simulink model "lab6sim"  (R2020a)
settings: Solver=VariableStepAuto  StartTime=0.0  StopTime=30  RelTol=1e-3
undefined symbols (not defined in the file or in its folder): den1, den2, den3, num1, num2, num3
settings Model: Creator=ariana  LastModifiedBy=ariana

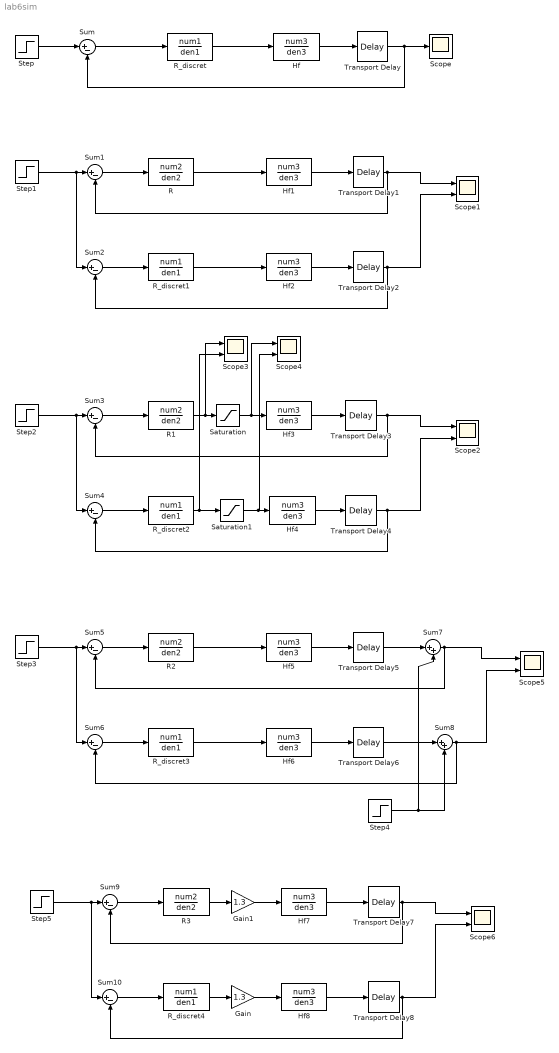
== system lab6sim ==
  Gain : Gain  Gain=1.3
  Gain1 : Gain  Gain=1.3
  Hf{,1..8} (9 alike) : TransferFcn  Numerator=num3  Denominator=den3
  R{,1..3} (4 alike) : TransferFcn  Numerator=num2  Denominator=den2
  R_discret{,1..4} (5 alike) : DiscreteTransferFcn  Numerator=num1  Denominator=den1  SampleTime=0.005
  Saturation : Saturate  UpperLimit=10  LowerLimit=0
  Saturation1 : Saturate  UpperLimit=10  LowerLimit=0
  Scope : Scope
  Scope{1..6} (6 alike) : Scope  NumInputPorts=2
  Step{,1..3,5} (5 alike) : Step  Time=0  After=20  SampleTime=0
  Step4 : Step  Time=10  After=5  SampleTime=0
  Sum{,1..6,9..10} (9 alike) : Sum  Inputs=|+-
  Sum7 : Sum  Inputs=|++
  Sum8 : Sum  Inputs=|++
  Transport Delay{,1..8} (9 alike) : TransportDelay  DelayTime=0.8
  wires:
  Step/1 -> Sum/1
  Sum/1 -> R_discret/1
  R_discret/1 -> Hf/1
  Hf/1 -> Transport Delay/1
  Transport Delay/1 -> Sum/2, Scope/1
  Step1/1 -> Sum2/1, Sum1/1
  Sum1/1 -> R/1
  Sum2/1 -> R_discret1/1
  R/1 -> Hf1/1
  R_discret1/1 -> Hf2/1
  Hf1/1 -> Transport Delay1/1
  Hf2/1 -> Transport Delay2/1
  Transport Delay1/1 -> Sum1/2, Scope1/1
  Transport Delay2/1 -> Sum2/2, Scope1/2
  Hf4/1 -> Transport Delay4/1
  Transport Delay3/1 -> Sum3/2, Scope2/1
  Transport Delay4/1 -> Sum4/2, Scope2/2
  Step2/1 -> Sum4/1, Sum3/1
  Hf3/1 -> Transport Delay3/1
  Sum3/1 -> R1/1
  R_discret2/1 -> Scope3/2, Saturation1/1
  Sum4/1 -> R_discret2/1
  R1/1 -> Scope3/1, Saturation/1
  Saturation1/1 -> Scope4/2, Hf4/1
  Saturation/1 -> Scope4/1, Hf3/1
  Sum5/1 -> R2/1
  Hf5/1 -> Transport Delay5/1
  Sum6/1 -> R_discret3/1
  Step3/1 -> Sum6/1, Sum5/1
  R2/1 -> Hf5/1
  R_discret3/1 -> Hf6/1
  Transport Delay5/1 -> Sum7/1
  Hf6/1 -> Transport Delay6/1
  Sum7/1 -> Sum5/2, Scope5/1
  Transport Delay6/1 -> Sum8/1
  Sum8/1 -> Sum6/2, Scope5/2
  Step4/1 -> Sum8/2, Sum7/2
  Sum9/1 -> R3/1
  Hf7/1 -> Transport Delay7/1
  Sum10/1 -> R_discret4/1
  Step5/1 -> Sum10/1, Sum9/1
  Transport Delay8/1 -> Sum10/2, Scope6/2
  Transport Delay7/1 -> Sum9/2, Scope6/1
  Hf8/1 -> Transport Delay8/1
  R3/1 -> Gain1/1
  Gain1/1 -> Hf7/1
  Gain/1 -> Hf8/1
  R_discret4/1 -> Gain/1
